simulink model "modelo_lqr_gab"  (R2023a)
settings: Solver=VariableStepAuto  StartTime=0.0  StopTime=10.0  RelTol=1e-3
undefined symbols (not defined in the file or in its folder): Ard, Brd, Crd, K, v_ic, x_ic
settings Model: Creator=gabri  LastModifiedBy=pinki
settings OptimizationCC: ReuseModelBlockBuffer=off

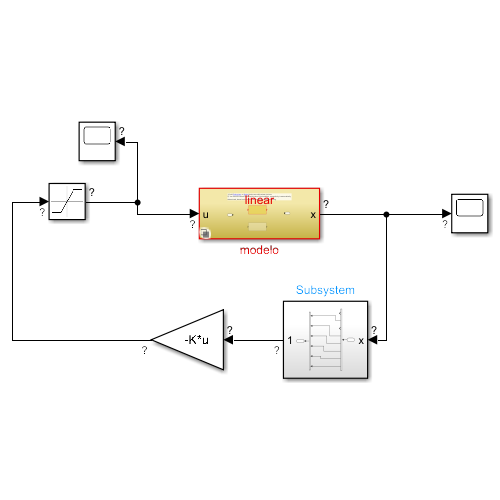
[thumbnail: Simulink's stored preview of the top-level diagram]
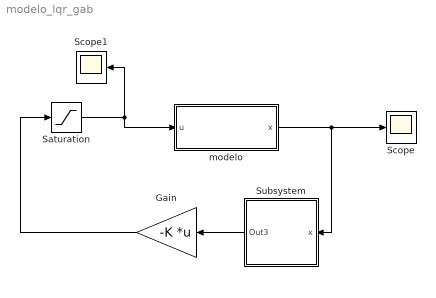
== system modelo_lqr_gab ==
  Gain : Gain  Gain=-K  Multiplication=Matrix(K*u)
  Saturation : Saturate  UpperLimit=1  LowerLimit=-1
  Scope : Scope
  Scope1 : Scope
  Subsystem : Subsystem
  modelo : Subsystem  Variant=on  VariantControlMode=label  LabelModeActiveChoice=false
  wires:
  Gain/1 -> Saturation/1
  Subsystem/1(Out3) -> Gain/1
  modelo/1(x) -> Scope/1, Subsystem/1(x)
  Saturation/1 -> modelo/1(u), Scope1/1

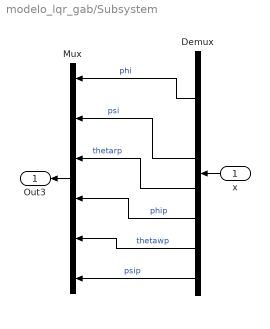
== system modelo_lqr_gab/Subsystem ==
  x : Inport
  Demux : Demux  Outputs=8
  Mux : Mux  Inputs=6
  Out3 : Outport
  wires:
  Demux/2 -> Mux/1  "phi"
  Demux/4 -> Mux/2  "psi"
  Demux/8 -> Mux/6  "psip"
  Demux/5 -> Mux/3  "thetarp"
  Demux/7 -> Mux/5  "thetawp"
  Demux/6 -> Mux/4  "phip"
  Mux/1 -> Out3/1
  x/1 -> Demux/1

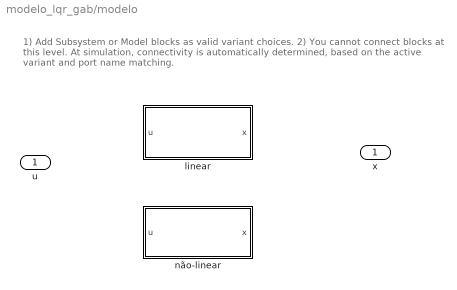
== system modelo_lqr_gab/modelo ==
  note: 1) Add Subsystem or Model blocks as valid variant choices.
      | 2) You cannot connect blocks at this level. At simulation, connectivity is automatically
      | determined, based on the active variant and port name matching.
  u : Inport
  linear : Subsystem  VariantControl=false
  não-linear : Subsystem  VariantControl=(default)
  x : Outport

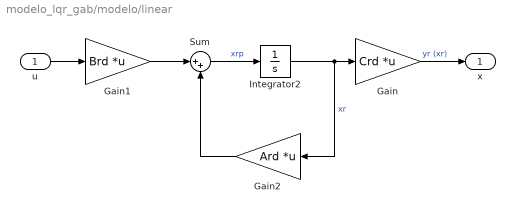
== system modelo_lqr_gab/modelo/linear ==
  u : Inport
  Gain : Gain  Gain=Crd  Multiplication=Matrix(K*u) (u vector)
  Gain1 : Gain  Gain=Brd  Multiplication=Matrix(K*u) (u vector)
  Gain2 : Gain  Gain=Ard  Multiplication=Matrix(K*u) (u vector)
  Integrator2 : Integrator  InitialCondition=x_ic
  Sum : Sum  Inputs=|++
  x : Outport
  wires:
  Gain2/1 -> Sum/2
  Gain1/1 -> Sum/1
  Integrator2/1 -> Gain2/1, Gain/1  "xr"
  u/1 -> Gain1/1
  Gain/1 -> x/1  "yr (xr)"
  Sum/1 -> Integrator2/1  "xrp"

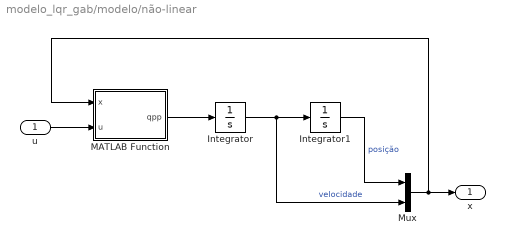
== system modelo_lqr_gab/modelo/não-linear ==
  u : Inport
  Integrator : Integrator  InitialCondition=v_ic
  Integrator1 : Integrator  InitialCondition=x_ic
  MATLAB Function : MATLAB Function  TreatAsAtomicUnit=on
  Mux : Mux  Inputs=2
  x : Outport
  wires:
  Integrator/1 -> Mux/2, Integrator1/1  "velocidade"
  MATLAB Function/1(qpp) -> Integrator/1
  u/1 -> MATLAB Function/2(u)
  Mux/1 -> MATLAB Function/1(x), x/1
  Integrator1/1 -> Mux/1  "posição"

== matlab function modelo_lqr_gab/modelo/não-linear/MATLAB Function ==
  data: x input; u input; qpp output
function qpp = fcn(x,u)

M = function_M(x(4));
V = function_V(x(6),x(4),x(8),x(5),x(7));
G = function_G(x(2),x(4));
P = function_P();

qpp = M^-1*(-V-G+P*u);
